simulink library "lib_Convection_ThinPlateCrossFlowHilpert"  (R2015a)
settings: Solver=ode45  StartTime=0.0  StopTime=10.0  RelTol=1e-3
libraries: simulink x7
settings Model: Creator=jlkratz  LastModifiedBy=jlkratz

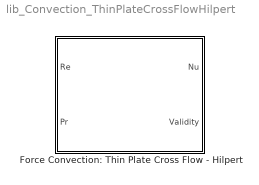
== system lib_Convection_ThinPlateCrossFlowHilpert ==
  Force Convection: Thin Plate Cross Flow - Hilpert : Subsystem  mask(TSAT: Thin Plate Cross Flow - Hilpert){FrontOrBack_M=Front side of the plate (side the flow is directed at)}
      mask help:
      | This block estimates the average Nusselt number of an external flow over an isothermal thin plate that is oriented perpendicular to the flow direction. The correlation employed was originally developed by Hilpert and has been modified to address non-circular cross-sectional shapes. It has an option to output the result for the front or back side of the thin plate. The Reynolds number (Re) should use the length of the plates cross-section as the characteristic length. The properties of the fluid should be evaluated at the film temperature. The correlation is subject to the following restrictions:
      |
      | Front side:
      | 10000 <= Re <= 50000
      | Pr >= 0.7
      |
      | Back side:
      | 7000 <= Re <= 80000
      | Pr >= 0.7
      |
      | Re is the Reynolds number and Pr is the Prandtl number. For more information see the block help menu.
      mask Help: web(which('Convection_TSAT_ThinPlateCrossFlowHilpert.html'),'-helpbrowser')
      mask TypeOptions FrontOrBack_M: Front side of the plate (side the flow is directed at) | Back side of the plate

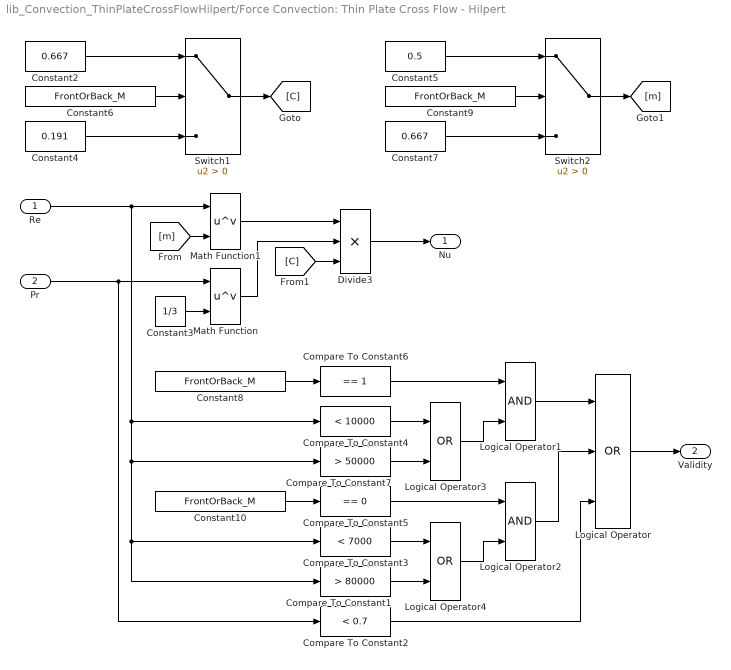
== system lib_Convection_ThinPlateCrossFlowHilpert/Force Convection: Thin Plate Cross Flow - Hilpert ==
  Re : Inport
  Pr : Inport  Port=2
  Compare To Constant1 : simulink/Logic and Bit Operations/Compare To Constant  relop=>  const=80000  OutDataTypeStr=boolean
  Compare To Constant2 : simulink/Logic and Bit Operations/Compare To Constant  relop=<  const=0.7  OutDataTypeStr=boolean
  Compare To Constant3 : simulink/Logic and Bit Operations/Compare To Constant  relop=<  const=7000  OutDataTypeStr=boolean
  Compare To Constant4 : simulink/Logic and Bit Operations/Compare To Constant  relop=<  const=10000  OutDataTypeStr=boolean
  Compare To Constant5 : simulink/Logic and Bit Operations/Compare To Constant  relop===  const=0  OutDataTypeStr=boolean
  Compare To Constant6 : simulink/Logic and Bit Operations/Compare To Constant  relop===  const=1  OutDataTypeStr=boolean
  Compare To Constant7 : simulink/Logic and Bit Operations/Compare To Constant  relop=>  const=50000  OutDataTypeStr=boolean
  Constant{6,8..10} (4 alike) : Constant  Value=FrontOrBack_M
  Constant2 : Constant  Value=0.667
  Constant3 : Constant  Value=1/3
  Constant4 : Constant  Value=0.191
  Constant5 : Constant  Value=0.5
  Constant7 : Constant  Value=0.667
  Divide3 : Product  Inputs=***
  Logical Operator : Logic  Operator=OR  Inputs=3  AllPortsSameDT=off  OutDataTypeStr=boolean
  Logical Operator1 : Logic  AllPortsSameDT=off  OutDataTypeStr=boolean
  Logical Operator2 : Logic  AllPortsSameDT=off  OutDataTypeStr=boolean
  Logical Operator3 : Logic  Operator=OR  AllPortsSameDT=off  OutDataTypeStr=boolean
  Logical Operator4 : Logic  Operator=OR  AllPortsSameDT=off  OutDataTypeStr=boolean
  Math Function : Math  Operator=pow  SaturateOnIntegerOverflow=on
  Math Function1 : Math  Operator=pow  SaturateOnIntegerOverflow=on
  Switch1 : Switch  Criteria=u2 > Threshold
  Switch2 : Switch  Criteria=u2 > Threshold
  Nu : Outport
  Validity : Outport  Port=2
  wires:
  Logical Operator4/1 -> Logical Operator2/2
  Logical Operator3/1 -> Logical Operator1/2
  Compare To Constant1/1 -> Logical Operator4/2
  Compare To Constant3/1 -> Logical Operator4/1
  Compare To Constant7/1 -> Logical Operator3/2
  Compare To Constant4/1 -> Logical Operator3/1
  Logical Operator/1 -> Validity/1
  Compare To Constant2/1 -> Logical Operator/3
  Logical Operator2/1 -> Logical Operator/2
  Logical Operator1/1 -> Logical Operator/1
  Compare To Constant5/1 -> Logical Operator2/1
  Compare To Constant6/1 -> Logical Operator1/1
  Constant10/1 -> Compare To Constant5/1
  Constant8/1 -> Compare To Constant6/1
  [C] -> Divide3/3
  Switch2/1 -> [m]
  Constant9/1 -> Switch2/2
  Constant7/1 -> Switch2/3
  Constant5/1 -> Switch2/1
  Switch1/1 -> [C]
  Constant6/1 -> Switch1/2
  Constant4/1 -> Switch1/3
  Constant2/1 -> Switch1/1
  Divide3/1 -> Nu/1
  Math Function1/1 -> Divide3/1
  Pr/1 -> Math Function/1, Compare To Constant2/1
  Re/1 -> Math Function1/1, Compare To Constant4/1, Compare To Constant1/1, Compare To Constant3/1, Compare To Constant7/1
  [m] -> Math Function1/2
  Constant3/1 -> Math Function/2
  Math Function/1 -> Divide3/2
